simulink model "gm_sampleModel1523_sub"  (R2023a)
settings: Solver=VariableStepAuto  StartTime=0.0  StopTime=10.0  RelTol=1e-3
libraries: hdlsllib x1
settings Model: Creator=user1  LastModifiedBy=user1
settings OptimizationCC: BlockReduction=off  ConditionallyExecuteInputs=off
settings DebuggingCC: InheritedTsInSrcMsg=none

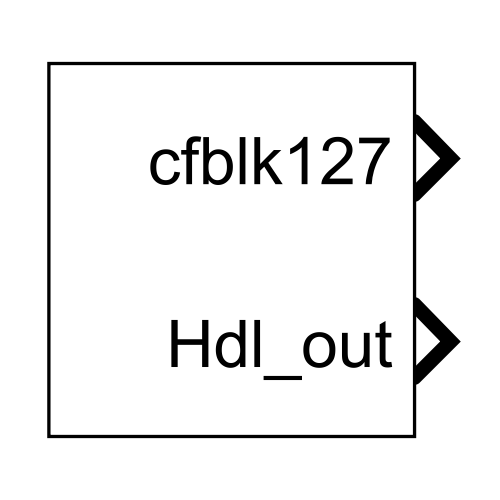
[thumbnail: Simulink's stored preview of the top-level diagram]
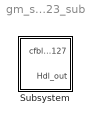
== system gm_sampleModel1523_sub ==
  Subsystem : Subsystem

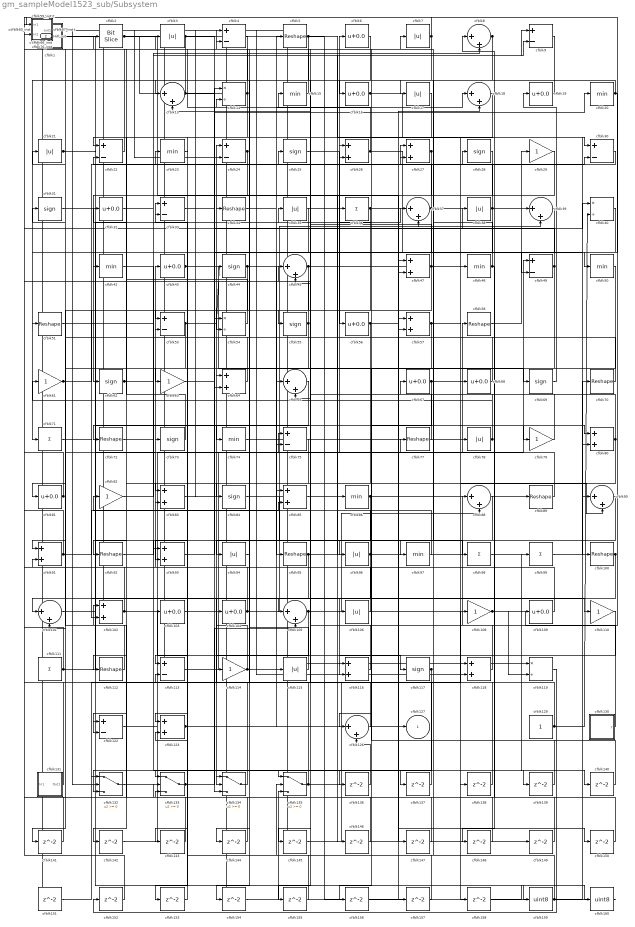
== system gm_sampleModel1523_sub/Subsystem ==
  cfblk1 : Subsystem  mask(Detect Rise Nonnegative){vinit=double(0), InputProcessing=Elements as channels (sample based), OutDataTypeStr=uint8}
      mask prompts: vinit "Simulink:masks:InitialCondition_MP"; InputProcessing "Simulink:masks:InputProcessing_MP"; OutDataTypeStr "Simulink:masks:OutputDataType_MP"
      mask help: Simulink:masks:DetectRiseNonnegative_MD
      mask init:
      | InputProcessing = 'Elements as channels (sample based)';
      | OutDataTypeStr = 'uint8';
      | vinit = double(0);
      mask TypeOptions InputProcessing: Simulink:masks:ColumnsAsChannelsFrameBased | Simulink:masks:ElementsAsChannelsSampleBased
      mask TypeOptions OutDataTypeStr: Simulink:masks:uint8 | Simulink:masks:boolean
      mask Display: fprintf('U >= 0\n&  NOT\nU/z >= 0')
  cfblk{5,34,51,58,70,72,77,89,92,95,100,112} (12 alike) : Reshape
  cfblk{8,13,18,37,39,45,65,88,90,101,105,126} (12 alike) : Sum  Inputs=|++  OutDataTypeStr=uint8
  cfblk{26..27,47,57,64,80,83,85,91,93,102,116,118,123} (14 alike) : Sum  OutDataTypeStr=uint8
  cfblk{6,16,19,32,43,56,67..68,81,103..104,109} (12 alike) : Bias  Bias=0.0  SaturateOnIntegerOverflow=off
  cfblk{3,7,17,21,35,38,78,94,96,106,115} (11 alike) : Abs  OutDataTypeStr=uint8  SaturateOnIntegerOverflow=off
  cfblk107_inst : Subsystem
  cfblk{29,61,63,79,82,108,110,114} (8 alike) : Gain  OutDataTypeStr=uint8
  cfblk10_inst : Subsystem
  cfblk{36,71,98..99,111} (5 alike) : Sum  Inputs=+  OutDataTypeStr=uint8
  cfblk{4,9,22,24,30,33,49,53,75,113,122} (11 alike) : Sum  Inputs=+-  OutDataTypeStr=uint8
  cfblk{25,28,31,44,55,62,69,73,84,117} (10 alike) : Signum
  cfblk{14,40,54,119} (4 alike) : Product  Inputs=*/  OutDataTypeStr=uint8  RndMeth=Zero  SaturateOnIntegerOverflow=on
  cfblk11_inst : Subsystem
  cfblk120_inst : Subsystem
  cfblk121_inst : Subsystem
  cfblk125_inst : Subsystem
  cfblk129 : Constant  OutDataTypeStr=uint8  SampleTime=-1
  cfblk12_inst : Subsystem
  cfblk130 : Subsystem  mask(Counter Limited){uplimit=double(7), tsamp=double(-1)}
      mask prompts: uplimit "Simulink:masks:UpperLimit_MP"; tsamp "Simulink:masks:SampleTime_MP"
      mask help: Simulink:masks:CounterLimited_MD
      mask init:
      | nbits = double(8);
      | tsamp = double(-1);
      | uplimit = double(7);
  cfblk131 : Subsystem
  cfblk{132..135} (4 alike) : Switch  OutDataTypeStr=uint8  SaturateOnIntegerOverflow=off  InputSameDT=off
  cfblk{136..158} (23 alike) : Delay  SampleTime=1
  cfblk{15,20,23,42,48,50,74,86,97} (9 alike) : MinMax  OutDataTypeStr=uint8
  cfblk159 : DataTypeConversion  OutDataTypeStr=uint8  SaturateOnIntegerOverflow=off  RndMeth=Floor
  cfblk160 : DataTypeConversion  OutDataTypeStr=uint8  SaturateOnIntegerOverflow=off  RndMeth=Floor
  cfblk2 : hdlsllib/Logic and Bit Operations/Bit Slice  lidx=7  ridx=0
  cfblk41_inst : Subsystem
  cfblk46_inst : Subsystem
  cfblk52_inst : Subsystem
  cfblk59_inst : Subsystem
  cfblk60_inst : Subsystem
  cfblk66_inst : Subsystem
  cfblk76_inst : Subsystem
  cfblk87_inst : Subsystem
  cfblk127 : Outport  OutDataTypeStr=uint8  SampleTime=1  VectorParamsAs1DForOutWhenUnconnected=off
  Hdl_out : Outport  Port=2  OutDataTypeStr=uint8  SampleTime=1
  wires:
  cfblk1/1(Y) -> cfblk159/1
  cfblk10_inst/1(out1) -> cfblk76_inst/2(in2), cfblk149/1
  cfblk100/1 -> cfblk116/2, cfblk101/1
  cfblk101/1 -> cfblk35/1
  cfblk102/1 -> cfblk66_inst/2(in2), cfblk117/1
  cfblk103/1 -> cfblk134/2
  cfblk104/1 -> cfblk43/1, cfblk39/2
  cfblk105/1 -> cfblk88/2, cfblk134/1
  cfblk106/1 -> cfblk24/1
  cfblk107_inst/1(out1) -> cfblk111/1
  cfblk108/1 -> cfblk12_inst/1(in1), cfblk119/2
  cfblk109/1 -> cfblk120_inst/2(in2)
  cfblk11_inst/1(out1) -> cfblk109/1, cfblk157/1
  cfblk110/1 -> cfblk116/1
  cfblk111/1 -> cfblk73/1, cfblk52_inst/2(in2)
  cfblk112/1 -> cfblk121_inst/1(in1)
  cfblk113/1 -> cfblk75/1
  cfblk114/1 -> cfblk5/1, cfblk34/1
  cfblk115/1 -> cfblk4/1
  cfblk116/1 -> cfblk45/1
  cfblk117/1 -> cfblk132/3, cfblk137/1
  cfblk118/1 -> cfblk46_inst/2(in2)
  cfblk119/1 -> cfblk152/1
  cfblk12_inst/1(out1) -> cfblk59_inst/1(in1), cfblk132/2, cfblk125_inst/2(in2)
  cfblk120_inst/1(out1) -> cfblk118/2, cfblk131/1(In1)
  cfblk121_inst/1(out1) -> cfblk119/1
  cfblk122/1 -> cfblk58/1
  cfblk123/1 -> cfblk65/1, cfblk47/1
  cfblk125_inst/1(out1) -> cfblk60_inst/2(in2), cfblk115/1
  cfblk126/1 -> cfblk33/1
  cfblk129/1 -> cfblk40/2, cfblk14/2
  cfblk13/1 -> cfblk87_inst/2(in2), cfblk75/2, cfblk47/2
  cfblk130/1(y) -> cfblk88/1
  cfblk131/1(Out1) -> cfblk125_inst/1(in1)
  cfblk132/1 -> cfblk6/1
  cfblk133/1 -> cfblk135/1, cfblk105/2
  cfblk134/1 -> cfblk120_inst/1(in1)
  cfblk135/1 -> cfblk64/1, cfblk108/1
  cfblk136/1 -> cfblk126/2
  cfblk137/1 -> cfblk65/2
  cfblk138/1 -> cfblk59_inst/2(in2)
  cfblk139/1 -> cfblk27/1
  cfblk14/1 -> cfblk4/2, cfblk22/1, Hdl_out/1
  cfblk140/1 -> cfblk12_inst/2(in2)
  cfblk141/1 -> cfblk60_inst/1(in1)
  cfblk142/1 -> cfblk49/1
  cfblk143/1 -> cfblk102/1
  cfblk144/1 -> cfblk133/3
  cfblk145/1 -> cfblk57/2
  cfblk146/1 -> cfblk132/1
  cfblk147/1 -> cfblk83/2
  cfblk148/1 -> cfblk133/2
  cfblk149/1 -> cfblk87_inst/1(in1)
  cfblk15/1 -> cfblk52_inst/1(in1)
  cfblk150/1 -> cfblk8/1
  cfblk151/1 -> cfblk118/1
  cfblk152/1 -> cfblk11_inst/2(in2)
  cfblk153/1 -> cfblk123/2
  cfblk154/1 -> cfblk135/3
  cfblk155/1 -> cfblk135/2
  cfblk156/1 -> cfblk18/2
  cfblk157/1 -> cfblk53/2
  cfblk158/1 -> cfblk160/1
  cfblk159/1 -> cfblk70/1, cfblk67/1, cfblk113/2
  cfblk16/1 -> cfblk80/2, cfblk68/1
  cfblk160/1 -> cfblk1/1(U)
  cfblk17/1 -> cfblk92/1
  cfblk18/1 -> cfblk83/1
  cfblk19/1 -> cfblk16/1
  cfblk2/1 -> cfblk147/1, cfblk146/1
  cfblk20/1 -> cfblk13/1, cfblk50/1
  cfblk21/1 -> cfblk79/1, cfblk98/1
  cfblk22/1 -> cfblk46_inst/1(in1)
  cfblk23/1 -> cfblk113/1
  cfblk24/1 -> cfblk62/1, cfblk63/1
  cfblk25/1 -> cfblk56/1
  cfblk26/1 -> cfblk76_inst/1(in1), cfblk100/1
  cfblk27/1 -> cfblk53/1, cfblk42/1
  cfblk28/1 -> cfblk142/1
  cfblk29/1 -> cfblk143/1
  cfblk3/1 -> cfblk49/2, cfblk41_inst/2(in2)
  cfblk30/1 -> cfblk22/2
  cfblk31/1 -> cfblk33/2
  cfblk32/1 -> cfblk26/1
  cfblk33/1 -> cfblk27/2
  cfblk34/1 -> cfblk30/2
  cfblk35/1 -> cfblk71/1
  cfblk36/1 -> cfblk102/2, cfblk158/1
  cfblk37/1 -> cfblk154/1, cfblk23/1
  cfblk38/1 -> cfblk7/1, cfblk153/1
  cfblk39/1 -> cfblk84/1
  cfblk4/1 -> cfblk51/1
  cfblk40/1 -> cfblk145/1
  cfblk41_inst/1(out1) -> cfblk39/1
  cfblk42/1 -> cfblk136/1
  cfblk43/1 -> cfblk85/1, cfblk69/1
  cfblk44/1 -> cfblk95/1, cfblk93/2
  cfblk45/1 -> cfblk91/1, cfblk40/1
  cfblk46_inst/1(out1) -> cfblk24/2, cfblk151/1
  cfblk47/1 -> cfblk54/2, cfblk15/1
  cfblk48/1 -> cfblk10_inst/1(in1), cfblk148/1
  cfblk49/1 -> cfblk134/3, cfblk11_inst/1(in1)
  cfblk5/1 -> cfblk64/2, cfblk30/1
  cfblk50/1 -> cfblk156/1
  cfblk51/1 -> cfblk8/2
  cfblk52_inst/1(out1) -> cfblk99/1
  cfblk53/1 -> cfblk44/1, cfblk122/2
  cfblk54/1 -> cfblk32/1
  cfblk55/1 -> cfblk81/1, cfblk66_inst/1(in1)
  cfblk56/1 -> cfblk37/2, cfblk155/1
  cfblk57/1 -> cfblk80/1, cfblk133/1
  cfblk58/1 -> cfblk29/1
  cfblk59_inst/1(out1) -> cfblk89/1, cfblk103/1, cfblk86/1
  cfblk6/1 -> cfblk104/1
  cfblk60_inst/1(out1) -> cfblk78/1
  cfblk61/1 -> cfblk28/1, cfblk141/1
  cfblk62/1 -> cfblk93/1, cfblk9/2, cfblk25/1
  cfblk63/1 -> cfblk38/1
  cfblk64/1 -> cfblk14/1
  cfblk65/1 -> cfblk72/1
  cfblk66_inst/1(out1) -> cfblk121_inst/2(in2)
  cfblk67/1 -> cfblk90/2, cfblk106/1
  cfblk68/1 -> cfblk21/1
  cfblk69/1 -> cfblk19/1
  cfblk7/1 -> cfblk55/1, cfblk41_inst/1(in1)
  cfblk70/1 -> cfblk57/1
  cfblk71/1 -> cfblk110/1
  cfblk72/1 -> cfblk74/1
  cfblk73/1 -> cfblk2/1
  cfblk74/1 -> cfblk18/1
  cfblk75/1 -> cfblk122/1
  cfblk76_inst/1(out1) -> cfblk127/1
  cfblk77/1 -> cfblk36/1
  cfblk78/1 -> cfblk13/2, cfblk61/1
  cfblk79/1 -> cfblk3/1
  cfblk8/1 -> cfblk45/2, cfblk17/1
  cfblk80/1 -> cfblk26/2, cfblk112/1
  cfblk81/1 -> cfblk107_inst/1(in1), cfblk10_inst/2(in2)
  cfblk82/1 -> cfblk37/1
  cfblk83/1 -> cfblk77/1
  cfblk84/1 -> cfblk138/1
  cfblk85/1 -> cfblk139/1
  cfblk86/1 -> cfblk126/1, cfblk105/1
  cfblk87_inst/1(out1) -> cfblk48/1
  cfblk88/1 -> cfblk94/1
  cfblk89/1 -> cfblk31/1
  cfblk9/1 -> cfblk97/1
  cfblk90/1 -> cfblk144/1
  cfblk91/1 -> cfblk85/2, cfblk107_inst/2(in2)
  cfblk92/1 -> cfblk96/1
  cfblk93/1 -> cfblk20/1
  cfblk94/1 -> cfblk114/1
  cfblk95/1 -> cfblk91/2, cfblk9/1, cfblk123/1
  cfblk96/1 -> cfblk101/2, cfblk54/1, cfblk150/1
  cfblk97/1 -> cfblk82/1
  cfblk98/1 -> cfblk140/1
  cfblk99/1 -> cfblk90/1

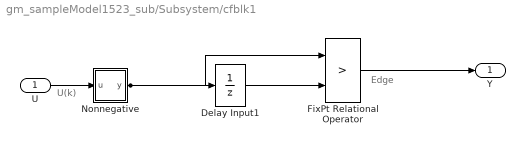
== system gm_sampleModel1523_sub/Subsystem/cfblk1 ==
  note: U(k)
  note: Edge
  U : Inport  OutDataTypeStr=uint8  SampleTime=1
  Delay Input1 : UnitDelay  Description=Store in Global RAM  DisableCoverage=on  InitialCondition=vinit  SampleTime=-1  HasFrameUpgradeWarning=on
  FixPt Relational Operator : RelationalOperator  Operator=>  OutDataTypeStr=fixdt(0, 8)  ZeroCross=off  InputSameDT=off
  Nonnegative : Subsystem  mask(Compare To Zero){relop=>=, OutDataTypeStr=boolean, ZeroCross=off}
      mask prompts: relop "Simulink:masks:Operator_MP"; OutDataTypeStr "Simulink:masks:OutputDataType_MP"; ZeroCross "Simulink:masks:EnableZerocrossingDetection_MP"
      mask help: Simulink:masks:CompareToZero_MD
      mask init:
      | OutDataTypeStr = 'boolean';
      | ZeroCross = 'off';
      | blkName = 'sampleModel1523_sub/Subsystem/cfblk1/Nonnegative';
      | relop = '>=';
      | setValue = 'boolean';
      mask TypeOptions relop: == | ~= | < | <= | >= | >
      mask TypeOptions OutDataTypeStr: Simulink:masks:uint8 | Simulink:masks:boolean
      mask Callback ZeroCross: sl('zeroCrossEnable', gcbh);
      mask Display: disp([relop,' 0'])
  Y : Outport  SampleTime=1
  wires:
  U/1 -> Nonnegative/1(u)
  Delay Input1/1 -> FixPt Relational Operator/2
  FixPt Relational Operator/1 -> Y/1
  Nonnegative/1(y) -> FixPt Relational Operator/1, Delay Input1/1

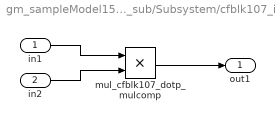
== system gm_sampleModel1523_sub/Subsystem/cfblk107_inst ==
  in1 : Inport  OutDataTypeStr=uint8  SampleTime=1
  in2 : Inport  Port=2  OutDataTypeStr=uint8  SampleTime=1
  mul_cfblk107_dotp_mulcomp : Product  Inputs=**  OutDataTypeStr=uint8  SampleTime=1
  out1 : Outport  OutDataTypeStr=uint8  SampleTime=1
  wires:
  in1/1 -> mul_cfblk107_dotp_mulcomp/1
  in2/1 -> mul_cfblk107_dotp_mulcomp/2
  mul_cfblk107_dotp_mulcomp/1 -> out1/1

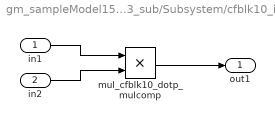
== system gm_sampleModel1523_sub/Subsystem/cfblk10_inst ==
  in1 : Inport  OutDataTypeStr=uint8  SampleTime=1
  in2 : Inport  Port=2  OutDataTypeStr=uint8  SampleTime=1
  mul_cfblk10_dotp_mulcomp : Product  Inputs=**  OutDataTypeStr=uint8  SampleTime=1
  out1 : Outport  OutDataTypeStr=uint8  SampleTime=1
  wires:
  in1/1 -> mul_cfblk10_dotp_mulcomp/1
  in2/1 -> mul_cfblk10_dotp_mulcomp/2
  mul_cfblk10_dotp_mulcomp/1 -> out1/1

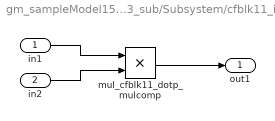
== system gm_sampleModel1523_sub/Subsystem/cfblk11_inst ==
  in1 : Inport  OutDataTypeStr=uint8  SampleTime=1
  in2 : Inport  Port=2  OutDataTypeStr=uint8  SampleTime=1
  mul_cfblk11_dotp_mulcomp : Product  Inputs=**  OutDataTypeStr=uint8  SampleTime=1
  out1 : Outport  OutDataTypeStr=uint8  SampleTime=1
  wires:
  in1/1 -> mul_cfblk11_dotp_mulcomp/1
  in2/1 -> mul_cfblk11_dotp_mulcomp/2
  mul_cfblk11_dotp_mulcomp/1 -> out1/1

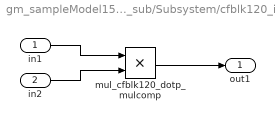
== system gm_sampleModel1523_sub/Subsystem/cfblk120_inst ==
  in1 : Inport  OutDataTypeStr=uint8  SampleTime=1
  in2 : Inport  Port=2  OutDataTypeStr=uint8  SampleTime=1
  mul_cfblk120_dotp_mulcomp : Product  Inputs=**  OutDataTypeStr=uint8  SampleTime=1
  out1 : Outport  OutDataTypeStr=uint8  SampleTime=1
  wires:
  in1/1 -> mul_cfblk120_dotp_mulcomp/1
  in2/1 -> mul_cfblk120_dotp_mulcomp/2
  mul_cfblk120_dotp_mulcomp/1 -> out1/1

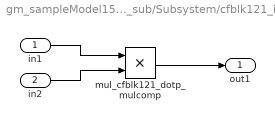
== system gm_sampleModel1523_sub/Subsystem/cfblk121_inst ==
  in1 : Inport  OutDataTypeStr=uint8  SampleTime=1
  in2 : Inport  Port=2  OutDataTypeStr=uint8  SampleTime=1
  mul_cfblk121_dotp_mulcomp : Product  Inputs=**  OutDataTypeStr=uint8  SampleTime=1
  out1 : Outport  OutDataTypeStr=uint8  SampleTime=1
  wires:
  in1/1 -> mul_cfblk121_dotp_mulcomp/1
  in2/1 -> mul_cfblk121_dotp_mulcomp/2
  mul_cfblk121_dotp_mulcomp/1 -> out1/1

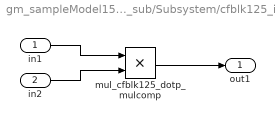
== system gm_sampleModel1523_sub/Subsystem/cfblk125_inst ==
  in1 : Inport  OutDataTypeStr=uint8  SampleTime=1
  in2 : Inport  Port=2  OutDataTypeStr=uint8  SampleTime=1
  mul_cfblk125_dotp_mulcomp : Product  Inputs=**  OutDataTypeStr=uint8  SampleTime=1
  out1 : Outport  OutDataTypeStr=uint8  SampleTime=1
  wires:
  in1/1 -> mul_cfblk125_dotp_mulcomp/1
  in2/1 -> mul_cfblk125_dotp_mulcomp/2
  mul_cfblk125_dotp_mulcomp/1 -> out1/1

== system gm_sampleModel1523_sub/Subsystem/cfblk12_inst ==
  in1 : Inport  OutDataTypeStr=uint8  SampleTime=1
  in2 : Inport  Port=2  OutDataTypeStr=uint8  SampleTime=1
  mul_cfblk12_dotp_mulcomp : Product  Inputs=**  OutDataTypeStr=uint8  SampleTime=1
  out1 : Outport  OutDataTypeStr=uint8  SampleTime=1
  wires:
  in1/1 -> mul_cfblk12_dotp_mulcomp/1
  in2/1 -> mul_cfblk12_dotp_mulcomp/2
  mul_cfblk12_dotp_mulcomp/1 -> out1/1

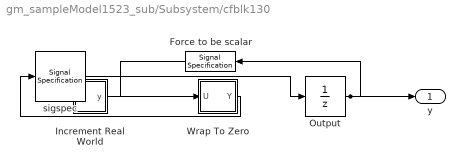
== system gm_sampleModel1523_sub/Subsystem/cfblk130 ==
  Force to be scalar : SignalSpecification  DisableCoverage=on  Dimensions=1
  Increment Real World : Subsystem  mask(Real World Value Increment){}
      mask help: Simulink:masks:RealWorldValueIncrement_MD
      mask Display: disp('V++')
  Output : UnitDelay  InitialCondition=0.0  SampleTime=tsamp  HasFrameUpgradeWarning=on
  Wrap To Zero : Subsystem  mask(Wrap To Zero){Threshold=double(7)}
      mask prompts: Threshold "Simulink:masks:Threshold_MP"
      mask help: Simulink:masks:WrapToZero_MD
  sigspec : SignalSpecification  OutDataTypeStr=uint8  Dimensions=1
  y : Outport  SampleTime=1
  wires:
  Force to be scalar/1 -> Increment Real World/1(u)
  Increment Real World/1(y) -> Wrap To Zero/1(U)
  Output/1 -> Force to be scalar/1, y/1
  Wrap To Zero/1(Y) -> sigspec/1
  sigspec/1 -> Output/1

== system gm_sampleModel1523_sub/Subsystem/cfblk131 ==
  In1 : Inport  OutDataTypeStr=uint8  PortDimensions=1  SampleTime=1
  Out1 : Outport  SampleTime=1
  wires:
  In1/1 -> Out1/1

== system gm_sampleModel1523_sub/Subsystem/cfblk41_inst ==
  in1 : Inport  OutDataTypeStr=uint8  SampleTime=1
  in2 : Inport  Port=2  OutDataTypeStr=uint8  SampleTime=1
  mul_cfblk41_dotp_mulcomp : Product  Inputs=**  OutDataTypeStr=uint8  SampleTime=1
  out1 : Outport  OutDataTypeStr=uint8  SampleTime=1
  wires:
  in1/1 -> mul_cfblk41_dotp_mulcomp/1
  in2/1 -> mul_cfblk41_dotp_mulcomp/2
  mul_cfblk41_dotp_mulcomp/1 -> out1/1

== system gm_sampleModel1523_sub/Subsystem/cfblk46_inst ==
  in1 : Inport  OutDataTypeStr=uint8  SampleTime=1
  in2 : Inport  Port=2  OutDataTypeStr=uint8  SampleTime=1
  mul_cfblk46_dotp_mulcomp : Product  Inputs=**  OutDataTypeStr=uint8  SampleTime=1
  out1 : Outport  OutDataTypeStr=uint8  SampleTime=1
  wires:
  in1/1 -> mul_cfblk46_dotp_mulcomp/1
  in2/1 -> mul_cfblk46_dotp_mulcomp/2
  mul_cfblk46_dotp_mulcomp/1 -> out1/1

== system gm_sampleModel1523_sub/Subsystem/cfblk52_inst ==
  in1 : Inport  OutDataTypeStr=uint8  SampleTime=1
  in2 : Inport  Port=2  OutDataTypeStr=uint8  SampleTime=1
  mul_cfblk52_dotp_mulcomp : Product  Inputs=**  OutDataTypeStr=uint8  SampleTime=1
  out1 : Outport  OutDataTypeStr=uint8  SampleTime=1
  wires:
  in1/1 -> mul_cfblk52_dotp_mulcomp/1
  in2/1 -> mul_cfblk52_dotp_mulcomp/2
  mul_cfblk52_dotp_mulcomp/1 -> out1/1

== system gm_sampleModel1523_sub/Subsystem/cfblk59_inst ==
  in1 : Inport  OutDataTypeStr=uint8  SampleTime=1
  in2 : Inport  Port=2  OutDataTypeStr=uint8  SampleTime=1
  mul_cfblk59_dotp_mulcomp : Product  Inputs=**  OutDataTypeStr=uint8  SampleTime=1
  out1 : Outport  OutDataTypeStr=uint8  SampleTime=1
  wires:
  in1/1 -> mul_cfblk59_dotp_mulcomp/1
  in2/1 -> mul_cfblk59_dotp_mulcomp/2
  mul_cfblk59_dotp_mulcomp/1 -> out1/1

== system gm_sampleModel1523_sub/Subsystem/cfblk60_inst ==
  in1 : Inport  OutDataTypeStr=uint8  SampleTime=1
  in2 : Inport  Port=2  OutDataTypeStr=uint8  SampleTime=1
  mul_cfblk60_dotp_mulcomp : Product  Inputs=**  OutDataTypeStr=uint8  SampleTime=1
  out1 : Outport  OutDataTypeStr=uint8  SampleTime=1
  wires:
  in1/1 -> mul_cfblk60_dotp_mulcomp/1
  in2/1 -> mul_cfblk60_dotp_mulcomp/2
  mul_cfblk60_dotp_mulcomp/1 -> out1/1

== system gm_sampleModel1523_sub/Subsystem/cfblk66_inst ==
  in1 : Inport  OutDataTypeStr=uint8  SampleTime=1
  in2 : Inport  Port=2  OutDataTypeStr=uint8  SampleTime=1
  mul_cfblk66_dotp_mulcomp : Product  Inputs=**  OutDataTypeStr=uint8  SampleTime=1
  out1 : Outport  OutDataTypeStr=uint8  SampleTime=1
  wires:
  in1/1 -> mul_cfblk66_dotp_mulcomp/1
  in2/1 -> mul_cfblk66_dotp_mulcomp/2
  mul_cfblk66_dotp_mulcomp/1 -> out1/1

== system gm_sampleModel1523_sub/Subsystem/cfblk76_inst ==
  in1 : Inport  OutDataTypeStr=uint8  SampleTime=1
  in2 : Inport  Port=2  OutDataTypeStr=uint8  SampleTime=1
  mul_cfblk76_dotp_mulcomp : Product  Inputs=**  OutDataTypeStr=uint8  SampleTime=1
  out1 : Outport  OutDataTypeStr=uint8  SampleTime=1
  wires:
  in1/1 -> mul_cfblk76_dotp_mulcomp/1
  in2/1 -> mul_cfblk76_dotp_mulcomp/2
  mul_cfblk76_dotp_mulcomp/1 -> out1/1

== system gm_sampleModel1523_sub/Subsystem/cfblk87_inst ==
  in1 : Inport  OutDataTypeStr=uint8  SampleTime=1
  in2 : Inport  Port=2  OutDataTypeStr=uint8  SampleTime=1
  mul_cfblk87_dotp_mulcomp : Product  Inputs=**  OutDataTypeStr=uint8  SampleTime=1
  out1 : Outport  OutDataTypeStr=uint8  SampleTime=1
  wires:
  in1/1 -> mul_cfblk87_dotp_mulcomp/1
  in2/1 -> mul_cfblk87_dotp_mulcomp/2
  mul_cfblk87_dotp_mulcomp/1 -> out1/1

== system gm_sampleModel1523_sub/Subsystem/cfblk1/Nonnegative ==
  u : Inport  OutDataTypeStr=uint8  SampleTime=1
  Compare : RelationalOperator  OutDataTypeStr=boolean  ZeroCross=off
  Constant : Constant  DisableCoverage=on  Value=0  OutDataTypeStr=Inherit: Inherit via back propagation  SampleTime=-1  PreserveConstantTs=on
  y : Outport  SampleTime=1
  wires:
  u/1 -> Compare/1
  Compare/1 -> y/1
  Constant/1 -> Compare/2

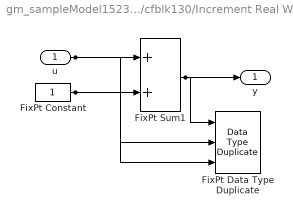
== system gm_sampleModel1523_sub/Subsystem/cfblk130/Increment Real World ==
  u : Inport  OutDataTypeStr=uint8  SampleTime=1
  FixPt Constant : Constant  DisableCoverage=on  OutDataTypeStr=Inherit: Inherit via back propagation  SampleTime=-1
  FixPt Data Type Duplicate : DataTypeDuplicate  DisableCoverage=on  NumInputPorts=3
  FixPt Sum1 : Sum  InputSameDT=on  OutDataTypeStr=Inherit: Inherit via back propagation  LockScale=on
  y : Outport  SampleTime=1
  wires:
  u/1 -> FixPt Sum1/1, FixPt Data Type Duplicate/2
  FixPt Constant/1 -> FixPt Sum1/2, FixPt Data Type Duplicate/3
  FixPt Sum1/1 -> FixPt Data Type Duplicate/1, y/1

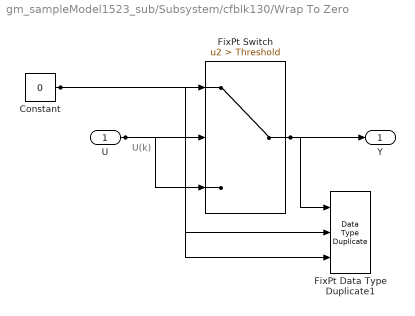
== system gm_sampleModel1523_sub/Subsystem/cfblk130/Wrap To Zero ==
  note: U(k)
  U : Inport  OutDataTypeStr=uint8  SampleTime=1
  Constant : Constant  DisableCoverage=on  Value=0  OutDataTypeStr=Inherit: Inherit via back propagation  SampleTime=-1
  FixPt Data Type Duplicate1 : DataTypeDuplicate  DisableCoverage=on  NumInputPorts=3
  FixPt Switch : Switch  Criteria=u2 > Threshold  Threshold=Threshold  OutDataTypeStr=Inherit: Inherit via back propagation  ZeroCross=off  SaturateOnIntegerOverflow=off  InputSameDT=off
  Y : Outport  SampleTime=1
  wires:
  U/1 -> FixPt Switch/3, FixPt Switch/2, FixPt Data Type Duplicate1/2
  Constant/1 -> FixPt Switch/1, FixPt Data Type Duplicate1/3
  FixPt Switch/1 -> FixPt Data Type Duplicate1/1, Y/1
